simulink model "3DoFManipulatorWithBLDCM_SIMULATION"  (R2023b)
settings: Solver=VariableStepAuto  StartTime=0.0  StopTime=10  MaxStep=1e-4  RelTol=1e-3
undefined symbols (not defined in the file): X, Y, Z
libraries: spsMosfetLib x18, sm_lib x11, nesl_utility x7, eeGeneralControl x6, spsDCVoltageSourceLib x3, spsGroundLib x3, spsThreePhaseSeriesRLCBranchLib x3, spsThreePhaseVIMeasurementLib x3, slpidlib x3, sps_lib x1
(part 1 of 3)
settings Model: Creator=nicog  LastModifiedBy=nicog

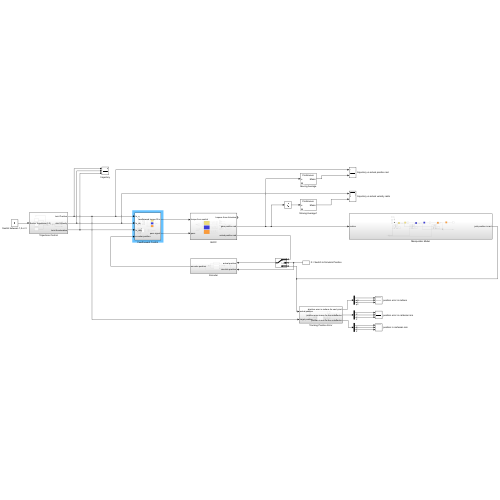
[thumbnail: Simulink's stored preview of the top-level diagram]
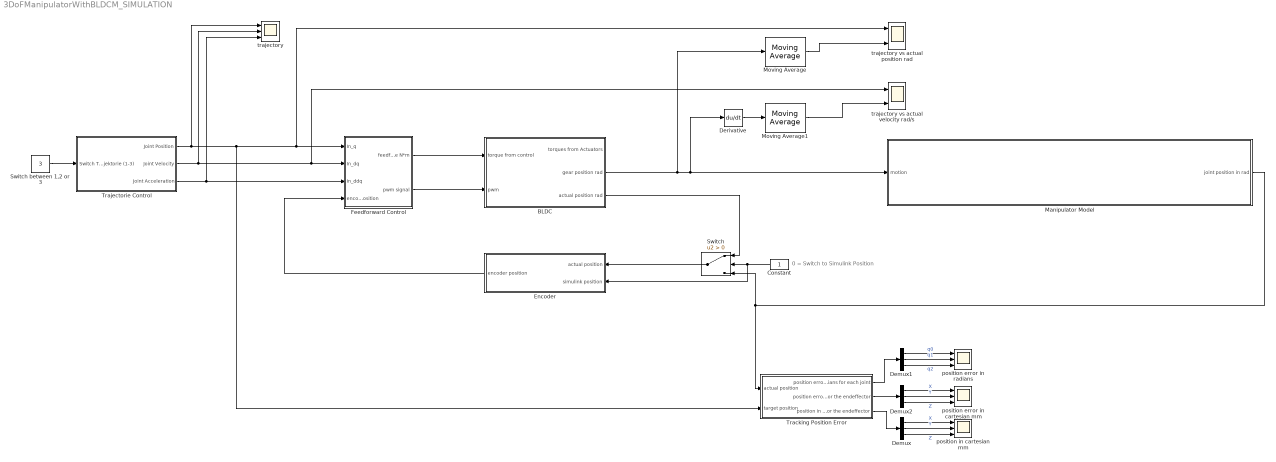
== system 3DoFManipulatorWithBLDCM_SIMULATION ==
  note: 0 = Switch to Simulink Position
  BLDC : Subsystem
  Constant : Constant
  Demux : Demux  Outputs=3
  Demux1 : Demux  Outputs=3
  Demux2 : Demux  Outputs=3
  Derivative : Derivative
  Encoder : Subsystem
  Feedforward Control : Subsystem
  Manipulator Model : Subsystem
  Moving Average : eeGeneralControl/Moving Average  VariantControl=Variant1  LabelModeActiveChoice=Continuous  f=60  x0=0  BufferSize=8192  Ts=0
      settings: LibrarySourceBlock=ee_sl_lib/General Control/Moving Average
  Moving Average1 : eeGeneralControl/Moving Average  VariantControl=Variant1  LabelModeActiveChoice=Continuous  f=60  x0=0  BufferSize=8192  Ts=0
      settings: LibrarySourceBlock=ee_sl_lib/General Control/Moving Average
  Switch : Switch  Criteria=u2 > Threshold  SaturateOnIntegerOverflow=off  InputSameDT=off
  Switch between 1,2 or 3 : Constant  Value=3
  Tracking Position Error : Subsystem
  Trajectorie Control : Subsystem
  position error in cartesian mm : Scope  NumInputPorts=3
  position error in radians : Scope  NumInputPorts=3
  position in cartesian mm : Scope  NumInputPorts=3
  trajectory : Scope  NumInputPorts=3
  trajectory vs actual position rad : Scope  NumInputPorts=2
  trajectory vs actual velocity rad/s : Scope  NumInputPorts=2
  wires:
  Trajectorie Control/2(Joint Velocity) -> trajectory/2, trajectory vs actual velocity rad/s/1, Feedforward Control/2(In_dq)
  Trajectorie Control/1(Joint Position) -> Tracking Position Error/2(target position), trajectory vs actual position rad/1, Feedforward Control/1(In_q), trajectory/1
  Trajectorie Control/3(Joint Acceleration) -> trajectory/3, Feedforward Control/3(In_ddq)
  Feedforward Control/1(feedforward torque N*m) -> BLDC/1(torque from control)
  Tracking Position Error/3(position in mm for the endeffector) -> Demux/1
  Switch between 1,2 or 3/1 -> Trajectorie Control/1(Switch Trajektorie (1-3))
  Demux/3 -> position in cartesian mm/3  "Z"
  Demux/2 -> position in cartesian mm/2  "Y"
  Demux/1 -> position in cartesian mm/1  "X"
  Tracking Position Error/1(position error in radians for each joint) -> Demux1/1
  Demux1/1 -> position error in radians/1  "q0"
  Demux1/2 -> position error in radians/2  "q1"
  Demux1/3 -> position error in radians/3  "q2"
  Demux2/1 -> position error in cartesian mm/1  "X"
  Demux2/2 -> position error in cartesian mm/2  "Y"
  Demux2/3 -> position error in cartesian mm/3  "Z"
  Tracking Position Error/2(position error in mm for the endeffector) -> Demux2/1
  BLDC/2(gear position rad) -> Moving Average/1, Derivative/1, Manipulator Model/1(motion)
  Switch/1 -> Encoder/1(actual position)
  Manipulator Model/1(joint position in rad) -> Tracking Position Error/1(actual position), Switch/3
  BLDC/3(actual position rad) -> Switch/1
  Constant/1 -> Encoder/2(simulink position), Switch/2
  Moving Average/1 -> trajectory vs actual position rad/2
  Moving Average1/1 -> trajectory vs actual velocity rad/s/2
  Derivative/1 -> Moving Average1/1
  Encoder/1(encoder position) -> Feedforward Control/4(encoder position)
  Feedforward Control/2(pwm signal) -> BLDC/2(pwm)

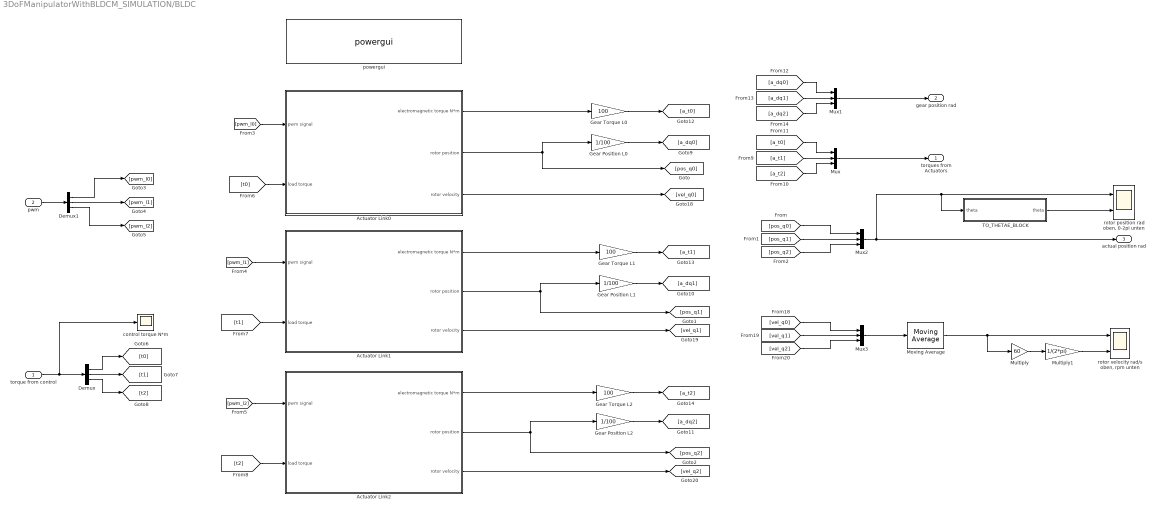
== system 3DoFManipulatorWithBLDCM_SIMULATION/BLDC ==
  torque from control : Inport
  pwm : Inport  Port=2
  Actuator Link0 : Subsystem
  Actuator Link1 : Subsystem
  Actuator Link2 : Subsystem
  Demux : Demux  Outputs=3
  Demux1 : Demux  Outputs=3
  Gear Position L0 : Gain  Gain=1/100
  Gear Position L1 : Gain  Gain=1/100
  Gear Position L2 : Gain  Gain=1/100
  Gear Torque L0 : Gain  Gain=100
  Gear Torque L1 : Gain  Gain=100
  Gear Torque L2 : Gain  Gain=100
  Moving Average : eeGeneralControl/Moving Average  VariantControl=Variant1  LabelModeActiveChoice=Continuous  f=30  x0=0  BufferSize=8192  Ts=0
      settings: LibrarySourceBlock=ee_sl_lib/General Control/Moving Average
  Multiply : Gain  Gain=60
  Multiply1 : Gain  Gain=1/(2*pi)
  Mux{,1..3} (4 alike) : Mux  Inputs=3
  TO_THETAE_BLOCK : MATLAB Function  TreatAsAtomicUnit=on
  control torque N*m : Scope
  powergui : sps_lib/powergui  Priority=1  SimulationMode=Discrete  SampleTime=1e-4  frequency=60  Iterations=50  frequencyindice=0  Pbase=100e6  ErrMax=1e-4  UnitsV=kV  UnitsW=MW  buscounter=0  FunctionMessages=off  echomessages=off  EnableUseOfTLC=off  CurrentSourceSwitches=off  DisableSnubberDevices=off  DisableRonSwitches=off  DisableVfSwitches=off  DisplayEquations=off  AutomaticDiscreteSolvers=off  SolverType=Tustin/Backward Euler (TBE)  Interpol=off  ExternalGateDelay=off  methode=off  Ts=100  x0status=blocks  SPID=on  SwTol=0  HookPort=off  NonlinearTolerance=1e-4  nMaxIteration=100  ContinueOnMaxIteration=off  RestoreLinks=warning  ResistiveCurrentMeasurement=off  Frange=[0:2:500]  Ylog=off  Xlog=on  ShowGrid=off  save=off  variable=ZData  structure=0  ZoomFFT=off  StartTime=0.0  cycles=1  DisplayStyle=1  fundamental=60  FreqAxis=off  MaxFrequency=1000  frequencyindicesteady=1  RmsSteady=1  display=off
  "rotor position rad oben, 0-2pi unten" : Scope  NumInputPorts=2
  "rotor velocity rad/s oben, rpm unten" : Scope  NumInputPorts=2
  torques from Actuators : Outport
  gear position rad : Outport  Port=2
  actual position rad : Outport  Port=3
  wires:
  torque from control/1 -> control torque N*m/1, Demux/1
  Actuator Link0/1(electromagnetic torque N*m) -> Gear Torque L0/1
  Actuator Link1/1(electromagnetic torque N*m) -> Gear Torque L1/1
  Actuator Link2/1(electromagnetic torque N*m) -> Gear Torque L2/1
  Mux1/1 -> gear position rad/1
  Mux2/1 -> TO_THETAE_BLOCK/1("theta "), "rotor position rad oben, 0-2pi unten"/1, actual position rad/1
  Mux/1 -> torques from Actuators/1
  Actuator Link0/2(rotor position) -> [pos_q0], Gear Position L0/1
  Actuator Link1/2(rotor position) -> [pos_q1], Gear Position L1/1
  Actuator Link2/2(rotor position) -> [pos_q2], Gear Position L2/1
  [pos_q0] -> Mux2/1
  [pos_q1] -> Mux2/2
  [pos_q2] -> Mux2/3
  Demux/1 -> [t0]
  Demux/2 -> [t1]
  Demux/3 -> [t2]
  [t0] -> Actuator Link0/2(load torque)
  Gear Position L0/1 -> [a_dq0]
  Gear Position L1/1 -> [a_dq1]
  Gear Position L2/1 -> [a_dq2]
  Gear Torque L0/1 -> [a_t0]
  Gear Torque L1/1 -> [a_t1]
  Gear Torque L2/1 -> [a_t2]
  [a_t0] -> Mux/1
  [a_t1] -> Mux/2
  [a_t2] -> Mux/3
  [a_dq0] -> Mux1/1
  [a_dq1] -> Mux1/2
  [a_dq2] -> Mux1/3
  [vel_q1] -> Mux3/2
  Mux3/1 -> Moving Average/1
  [vel_q2] -> Mux3/3
  [vel_q0] -> Mux3/1
  Multiply/1 -> Multiply1/1
  Moving Average/1 -> Multiply/1, "rotor velocity rad/s oben, rpm unten"/1
  Multiply1/1 -> "rotor velocity rad/s oben, rpm unten"/2
  TO_THETAE_BLOCK/1(theta) -> "rotor position rad oben, 0-2pi unten"/2
  Actuator Link0/3(rotor velocity) -> [vel_q0]
  Actuator Link1/3(rotor velocity) -> [vel_q1]
  Actuator Link2/3(rotor velocity) -> [vel_q2]
  [t1] -> Actuator Link1/2(load torque)
  pwm/1 -> Demux1/1
  Demux1/1 -> [pwm_l0]
  Demux1/2 -> [pwm_l1]
  Demux1/3 -> [pwm_l2]
  [pwm_l0] -> Actuator Link0/1(pwm signal)
  [pwm_l1] -> Actuator Link1/1(pwm signal)
  [pwm_l2] -> Actuator Link2/1(pwm signal)
  [t2] -> Actuator Link2/2(load torque)

== system 3DoFManipulatorWithBLDCM_SIMULATION/Encoder ==
  actual position : Inport
  simulink position : Inport  Port=2
  Demux : Demux  Outputs=3
  ENCODER_BLOCK_L0 : MATLAB Function  TreatAsAtomicUnit=on  SystemSampleTime=1e-4
  ENCODER_BLOCK_L1 : MATLAB Function  TreatAsAtomicUnit=on  SystemSampleTime=1e-4
  ENCODER_BLOCK_L2 : MATLAB Function  TreatAsAtomicUnit=on  SystemSampleTime=1e-4
  Mux : Mux  Inputs=3
  Switch : Switch  Criteria=u2 > Threshold  SaturateOnIntegerOverflow=off  InputSameDT=off
  encoder position : Outport
  wires:
  Demux/1 -> ENCODER_BLOCK_L0/1(actual_position)
  Demux/2 -> ENCODER_BLOCK_L1/1(actual_position)
  Demux/3 -> ENCODER_BLOCK_L2/1(actual_position)
  ENCODER_BLOCK_L1/1(encoder_output) -> Mux/2
  ENCODER_BLOCK_L2/1(encoder_output) -> Mux/3
  ENCODER_BLOCK_L0/1(encoder_output) -> Mux/1
  simulink position/1 -> Switch/2
  Mux/1 -> Switch/1
  actual position/1 -> Demux/1, Switch/3
  Switch/1 -> encoder position/1

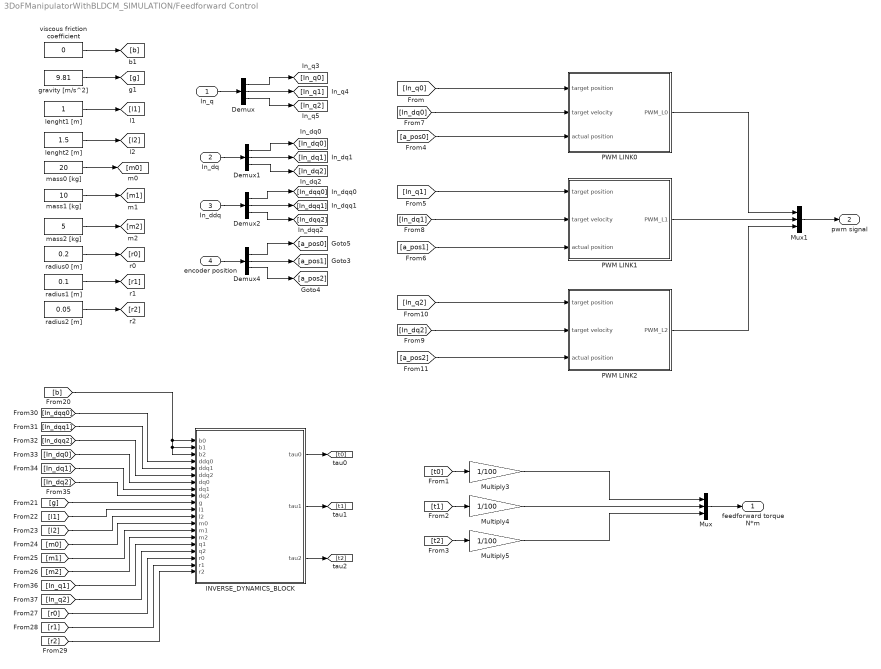
== system 3DoFManipulatorWithBLDCM_SIMULATION/Feedforward Control ==
  In_q : Inport
  In_dq : Inport  Port=2
  In_ddq : Inport  Port=3
  encoder position : Inport  Port=4
  Demux{,1..2,4} (4 alike) : Demux  Outputs=3
  INVERSE_DYNAMICS_BLOCK : MATLAB Function  TreatAsAtomicUnit=on
  Multiply3 : Gain  Gain=1/100
  Multiply4 : Gain  Gain=1/100
  Multiply5 : Gain  Gain=1/100
  Mux : Mux  Inputs=3
  Mux1 : Mux  Inputs=3
  PWM LINK0 : Subsystem
  PWM LINK1 : Subsystem
  PWM LINK2 : Subsystem
  "gravity [m/s^2] " : Constant  Value=9.81
  lenght1 [m] : Constant
  lenght2 [m] : Constant  Value=1.5
  mass0 [kg] : Constant  Value=20
  mass1 [kg] : Constant  Value=10
  mass2 [kg] : Constant  Value=5
  radius0 [m] : Constant  Value=0.2
  radius1 [m] : Constant  Value=0.1
  radius2 [m] : Constant  Value=0.05
  viscous friction coefficient : Constant  Value=0
  feedforward torque N*m : Outport
  pwm signal : Outport  Port=2
  wires:
  [r2] -> INVERSE_DYNAMICS_BLOCK/20(r2)
  [g] -> INVERSE_DYNAMICS_BLOCK/10(g)
  [r0] -> INVERSE_DYNAMICS_BLOCK/18(r0)
  [b] -> INVERSE_DYNAMICS_BLOCK/2(b1), INVERSE_DYNAMICS_BLOCK/3(b2), INVERSE_DYNAMICS_BLOCK/1(b0)
  [l1] -> INVERSE_DYNAMICS_BLOCK/11(l1)
  [m1] -> INVERSE_DYNAMICS_BLOCK/14(m1)
  [m2] -> INVERSE_DYNAMICS_BLOCK/15(m2)
  [m0] -> INVERSE_DYNAMICS_BLOCK/13(m0)
  [r1] -> INVERSE_DYNAMICS_BLOCK/19(r1)
  [l2] -> INVERSE_DYNAMICS_BLOCK/12(l2)
  In_q/1 -> Demux/1
  In_dq/1 -> Demux1/1
  In_ddq/1 -> Demux2/1
  Mux/1 -> feedforward torque N*m/1
  radius0 [m]/1 -> [r0]
  radius2 [m]/1 -> [r2]
  lenght2 [m]/1 -> [l2]
  viscous friction coefficient/1 -> [b]
  radius1 [m]/1 -> [r1]
  lenght1 [m]/1 -> [l1]
  mass0 [kg]/1 -> [m0]
  mass1 [kg]/1 -> [m1]
  mass2 [kg]/1 -> [m2]
  "gravity [m/s^2] "/1 -> [g]
  INVERSE_DYNAMICS_BLOCK/3(tau2) -> [t2]
  [t0] -> Multiply3/1
  [t1] -> Multiply4/1
  [t2] -> Multiply5/1
  Demux2/1 -> [In_dqq0]
  Demux2/2 -> [In_dqq1]
  Demux2/3 -> [In_dqq2]
  Demux1/2 -> [In_dq1]
  Demux1/1 -> [In_dq0]
  Demux1/3 -> [In_dq2]
  Demux/2 -> [In_q1]
  Demux/1 -> [In_q0]
  Demux/3 -> [In_q2]
  [In_dqq0] -> INVERSE_DYNAMICS_BLOCK/4(ddq0)
  [In_dqq1] -> INVERSE_DYNAMICS_BLOCK/5(ddq1)
  [In_dqq2] -> INVERSE_DYNAMICS_BLOCK/6(ddq2)
  [In_dq0] -> INVERSE_DYNAMICS_BLOCK/7(dq0)
  [In_dq1] -> INVERSE_DYNAMICS_BLOCK/8(dq1)
  [In_dq2] -> INVERSE_DYNAMICS_BLOCK/9(dq2)
  [In_q1] -> INVERSE_DYNAMICS_BLOCK/16(q1)
  [In_q2] -> INVERSE_DYNAMICS_BLOCK/17(q2)
  INVERSE_DYNAMICS_BLOCK/2(tau1) -> [t1]
  INVERSE_DYNAMICS_BLOCK/1(tau0) -> [t0]
  Multiply3/1 -> Mux/1
  Multiply4/1 -> Mux/2
  Multiply5/1 -> Mux/3
  PWM LINK0/1(PWM_L0) -> Mux1/1
  Mux1/1 -> pwm signal/1
  [In_q1] -> PWM LINK1/1(target position)
  PWM LINK1/1(PWM_L1) -> Mux1/2
  [a_pos1] -> PWM LINK1/3(actual position)
  [a_pos0] -> PWM LINK0/3(actual position)
  Demux4/2 -> [a_pos1]
  [In_q0] -> PWM LINK0/1(target position)
  Demux4/3 -> [a_pos2]
  [a_pos2] -> PWM LINK2/3(actual position)
  Demux4/1 -> [a_pos0]
  [In_q2] -> PWM LINK2/1(target position)
  encoder position/1 -> Demux4/1
  PWM LINK2/1(PWM_L2) -> Mux1/3
  [In_dq0] -> PWM LINK0/2(target velocity)
  [In_dq1] -> PWM LINK1/2(target velocity)
  [In_dq2] -> PWM LINK2/2(target velocity)

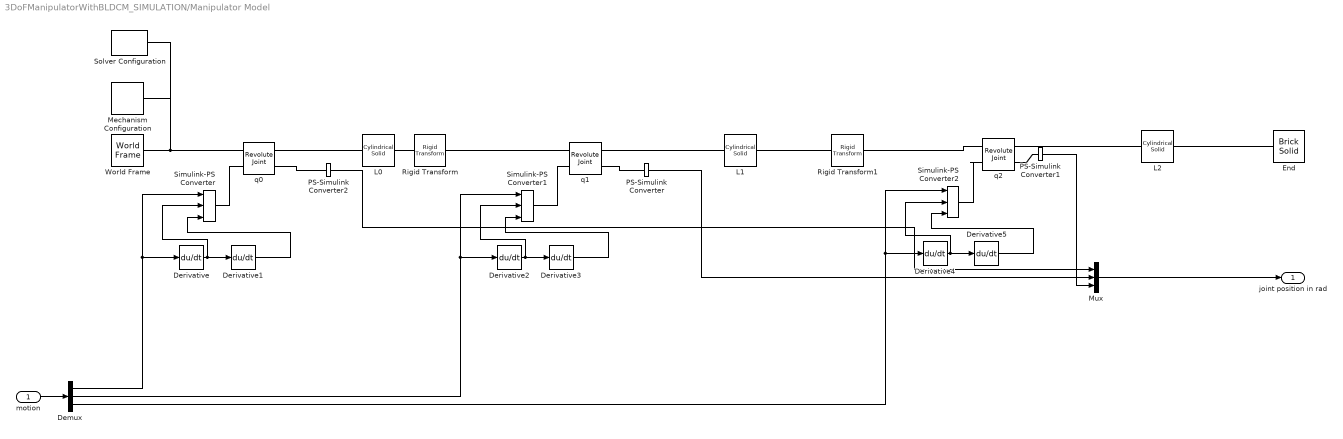
== system 3DoFManipulatorWithBLDCM_SIMULATION/Manipulator Model ==
  motion : Inport
  " L1" : sm_lib/Body Elements/Cylindrical Solid  GraphicAmbientColor=[0.15 0.15 0.15 1.0]  BasedOnType=Density  CenterOfMass=[0 0 0]  CenterOfMassUnits=m  GraphicDiffuseColor=[0.0 0.0 1.0]  CylinderLength=1  CylinderLengthUnits=m  CylinderRadius=0.1  CylinderRadiusUnits=m  Density=1000  DensityUnits=kg/m^3  DoExposeReferenceFrame=off  GraphicEmissiveColor=[0.0 0.0 0.0 1.0]  ExportEntireGeometry=off  SerializedFrames=<Frames><Frame><Id>Frame1</Id><Value><Name>F1</Name><Origin><Source>GeometricFeature</Source><FeatureName>bottom surface</FeatureName></Origin><PrimaryAxis><DefinedDirection>+X</DefinedDirection><Source>ReferenceFrame</Source><SourceDirection>+Z</SourceDirection><FeatureName></FeatureName></PrimaryAxis><SecondaryAxis><DefinedDirection>+Y</DefinedDirection><Source>ReferenceFrame</Source><SourceDirection>+X</SourceDirection><FeatureName></FeatureName></SecondaryAxis></Value></Frame><Frame><Id>Frame2</Id><Value><Name>F2</Name><Origin><Source>GeometricFeature</Source><FeatureName>top surface</FeatureName></Origin><PrimaryAxis><DefinedDirection>+X</DefinedDirection><Source>ReferenceFrame</Source><SourceDirection>+Z</SourceDirection><FeatureName></FeatureName></PrimaryAxis><SecondaryAxis><DefinedDirection>+Y</DefinedDirection><Source>ReferenceFrame</Source><SourceDirection>+X</SourceDirection><FeatureName></FeatureName></SecondaryAxis></Value></Frame></Frames>  MarkerShape=Sphere  MarkerSize=10  GraphicType=FromGeometry  InertiaType=PointMass  Mass=10  MassUnits=kg  MomentsOfInertia=[1 1 1]  MomentsOfInertiaUnits=kg*m^2  GraphicOpacity=1.0  ProductsOfInertia=[0 0 0]  ProductsOfInertiaUnits=kg*m^2  GraphicShininess=75  GraphicSpecularColor=[0.5 0.5 0.5 1.0]  GraphicVisPropType=SimpleVisualProperties
  Demux : Demux  Outputs=3
  Derivative{,1..5} (6 alike) : Derivative
  End : sm_lib/Body Elements/Brick Solid  GraphicAmbientColor=[0.15 0.15 0.15 1.0]  BasedOnType=Density  BrickDimensions=[1 1 1]  BrickDimensionsUnits=cm  CenterOfMass=[0 0 0]  CenterOfMassUnits=m  GraphicDiffuseColor=[1.0 0.0 0.4]  Density=1000  DensityUnits=kg/m^3  DoExposeReferenceFrame=on  GraphicEmissiveColor=[0.0 0.0 0.0 1.0]  ExportEntireGeometry=off  SerializedFrames=<Frames/>  MarkerShape=Sphere  MarkerSize=10  GraphicType=FromGeometry  InertiaType=PointMass  Mass=1  MassUnits=g  MomentsOfInertia=[1 1 1]  MomentsOfInertiaUnits=kg*m^2  GraphicOpacity=1.0  ProductsOfInertia=[0 0 0]  ProductsOfInertiaUnits=kg*m^2  GraphicShininess=75  GraphicSpecularColor=[0.5 0.5 0.5 1.0]  GraphicVisPropType=SimpleVisualProperties
  L0 : sm_lib/Body Elements/Cylindrical Solid  GraphicAmbientColor=[0.15 0.15 0.15 1.0]  BasedOnType=Density  CenterOfMass=[0 0 0]  CenterOfMassUnits=m  GraphicDiffuseColor=[1.0 1.0 0.0]  CylinderLength=0.5  CylinderLengthUnits=m  CylinderRadius=0.2  CylinderRadiusUnits=m  Density=1000  DensityUnits=kg/m^3  DoExposeReferenceFrame=off  GraphicEmissiveColor=[0.0 0.0 0.0 1.0]  ExportEntireGeometry=off  SerializedFrames=<Frames><Frame><Id>Frame1</Id><Value><Name>Bottom</Name><Origin><Source>GeometricFeature</Source><FeatureName>bottom surface</FeatureName></Origin><PrimaryAxis><DefinedDirection>+Z</DefinedDirection><Source>ReferenceFrame</Source><SourceDirection>+Z</SourceDirection><FeatureName></FeatureName></PrimaryAxis><SecondaryAxis><DefinedDirection>+X</DefinedDirection><Source>ReferenceFrame</Source><SourceDirection>+X</SourceDirection><FeatureName></FeatureName></SecondaryAxis></Value></Frame><Frame><Id>Frame2</Id><Value><Name>Top</Name><Origin><Source>GeometricFeature</Source><FeatureName>top surface</FeatureName></Origin><PrimaryAxis><DefinedDirection>+Z</DefinedDirection><Source>ReferenceFrame</Source><SourceDirection>+Z</SourceDirection><FeatureName></FeatureName></PrimaryAxis><SecondaryAxis><DefinedDirection>+X</DefinedDirection><Source>ReferenceFrame</Source><SourceDirection>+X</SourceDirection><FeatureName></FeatureName></SecondaryAxis></Value></Frame></Frames>  MarkerShape=Sphere  MarkerSize=10  GraphicType=FromGeometry  InertiaType=PointMass  Mass=20  MassUnits=kg  MomentsOfInertia=[1 1 1]  MomentsOfInertiaUnits=kg*m^2  GraphicOpacity=1.0  ProductsOfInertia=[0 0 0]  ProductsOfInertiaUnits=kg*m^2  GraphicShininess=75  GraphicSpecularColor=[0.5 0.5 0.5 1.0]  GraphicVisPropType=SimpleVisualProperties
  L2 : sm_lib/Body Elements/Cylindrical Solid  GraphicAmbientColor=[0.15 0.15 0.15 1.0]  BasedOnType=Density  CenterOfMass=[0 0 0]  CenterOfMassUnits=m  GraphicDiffuseColor=[1.0 0.6 0.0]  CylinderLength=1.5  CylinderLengthUnits=m  CylinderRadius=0.05  CylinderRadiusUnits=m  Density=1000  DensityUnits=kg/m^3  DoExposeReferenceFrame=off  GraphicEmissiveColor=[0.0 0.0 0.0 1.0]  ExportEntireGeometry=off  SerializedFrames=<Frames><Frame><Id>Frame1</Id><Value><Name>F1</Name><Origin><Source>GeometricFeature</Source><FeatureName>bottom surface</FeatureName></Origin><PrimaryAxis><DefinedDirection>+X</DefinedDirection><Source>ReferenceFrame</Source><SourceDirection>+Z</SourceDirection><FeatureName></FeatureName></PrimaryAxis><SecondaryAxis><DefinedDirection>+Y</DefinedDirection><Source>ReferenceFrame</Source><SourceDirection>+X</SourceDirection><FeatureName></FeatureName></SecondaryAxis></Value></Frame><Frame><Id>Frame2</Id><Value><Name>F2</Name><Origin><Source>GeometricFeature</Source><FeatureName>top surface</FeatureName></Origin><PrimaryAxis><DefinedDirection>+X</DefinedDirection><Source>ReferenceFrame</Source><SourceDirection>+Z</SourceDirection><FeatureName></FeatureName></PrimaryAxis><SecondaryAxis><DefinedDirection>+Y</DefinedDirection><Source>ReferenceFrame</Source><SourceDirection>+X</SourceDirection><FeatureName></FeatureName></SecondaryAxis></Value></Frame></Frames>  MarkerShape=Sphere  MarkerSize=10  GraphicType=FromGeometry  InertiaType=PointMass  Mass=5  MassUnits=kg  MomentsOfInertia=[1 1 1]  MomentsOfInertiaUnits=kg*m^2  GraphicOpacity=1.0  ProductsOfInertia=[0 0 0]  ProductsOfInertiaUnits=kg*m^2  GraphicShininess=75  GraphicSpecularColor=[0.5 0.5 0.5 1.0]  GraphicVisPropType=SimpleVisualProperties
  Mechanism Configuration : sm_lib/Utilities/Mechanism Configuration  UniformGravity=Constant  GravityVector=[0 0 -9.80665]  GravityVectorUnits=m/s^2  LinearizationDelta=0.001  JointModeTransitionNonlinearIterations=2
  Mux : Mux  Inputs=3
  PS-Simulink Converter : nesl_utility/PS-Simulink Converter  PhysicalDomain=network_engine_domain  SubClassName=ps_output  LeftPortType=input  RightPortType=output  PseudoPeriodic=off  Frequencies=[]  VectorFormat=inherit  Unit=inherit  AffineConversion=off
  PS-Simulink Converter1 : nesl_utility/PS-Simulink Converter  PhysicalDomain=network_engine_domain  SubClassName=ps_output  LeftPortType=input  RightPortType=output  PseudoPeriodic=off  Frequencies=[]  VectorFormat=inherit  Unit=inherit  AffineConversion=off
  PS-Simulink Converter2 : nesl_utility/PS-Simulink Converter  PhysicalDomain=network_engine_domain  SubClassName=ps_output  LeftPortType=input  RightPortType=output  PseudoPeriodic=off  Frequencies=[]  VectorFormat=inherit  Unit=inherit  AffineConversion=off
  Rigid Transform : sm_lib/Frames and Transforms/Rigid Transform  TranslationMethod=None  TranslationStandardOffset=0  TranslationStandardOffsetUnits=m  TranslationStandardAxis=+Z  TranslationCartesianOffset=[0 0 0]  TranslationCartesianOffsetUnits=m  TranslationROffset=0  TranslationROffsetUnits=m  TranslationZOffset=0  TranslationZOffsetUnits=m  TranslationThetaOffset=0  TranslationThetaOffsetUnits=deg  RotationMethod=RotationSequence  RotationAngleUnits=rad  RotationStandardAxis=+X  RotationAngle=pi/2  RotationArbitraryAxis=[0 0 1]  FollAlignAxisA=+X  BaseAlignAxisA=+Y  FollAlignAxisB=+Y  BaseAlignAxisB=+Z  RotationSequenceAxes=FollowerAxes  RotationSequence=XZX  RotationSequenceAngles=[90 140 0]  RotationSequenceAnglesUnits=deg  RotationMatrix=[1 0 0; 0 1 0; 0 0 1]  Quaternion=[1 0 0 0]
  Rigid Transform1 : sm_lib/Frames and Transforms/Rigid Transform  TranslationMethod=None  TranslationStandardOffset=0  TranslationStandardOffsetUnits=m  TranslationStandardAxis=+Z  TranslationCartesianOffset=[0 0 0]  TranslationCartesianOffsetUnits=m  TranslationROffset=0  TranslationROffsetUnits=m  TranslationZOffset=0  TranslationZOffsetUnits=m  TranslationThetaOffset=0  TranslationThetaOffsetUnits=deg  RotationMethod=RotationSequence  RotationAngleUnits=rad  RotationStandardAxis=+X  RotationAngle=pi/2  RotationArbitraryAxis=[0 0 1]  FollAlignAxisA=+X  BaseAlignAxisA=+Y  FollAlignAxisB=+Y  BaseAlignAxisB=+Z  RotationSequenceAxes=FollowerAxes  RotationSequence=ZXY  RotationSequenceAngles=[-140 0 0]  RotationSequenceAnglesUnits=deg  RotationMatrix=[1 0 0; 0 1 0; 0 0 1]  Quaternion=[1 0 0 0]
  Simulink-PS Converter : nesl_utility/Simulink-PS Converter  PhysicalDomain=network_engine_domain  SubClassName=ps_input  LeftPortType=input  RightPortType=output  PseudoPeriodic=off  Frequencies=[]  NoiseDistribution=none  NoiseParameters=[]  Unit=rad  AffineConversion=off  FilteringAndDerivatives=provide  SimscapeFilterOrder=2  InputFilterTimeConstant=0.001  UdotUserProvided=2
  Simulink-PS Converter1 : nesl_utility/Simulink-PS Converter  PhysicalDomain=network_engine_domain  SubClassName=ps_input  LeftPortType=input  RightPortType=output  PseudoPeriodic=off  Frequencies=[]  NoiseDistribution=none  NoiseParameters=[]  Unit=rad  AffineConversion=off  FilteringAndDerivatives=provide  SimscapeFilterOrder=2  InputFilterTimeConstant=0.001  UdotUserProvided=2
  Simulink-PS Converter2 : nesl_utility/Simulink-PS Converter  PhysicalDomain=network_engine_domain  SubClassName=ps_input  LeftPortType=input  RightPortType=output  PseudoPeriodic=off  Frequencies=[]  NoiseDistribution=none  NoiseParameters=[]  Unit=rad  AffineConversion=off  FilteringAndDerivatives=provide  SimscapeFilterOrder=2  InputFilterTimeConstant=0.001  UdotUserProvided=2
  Solver Configuration : nesl_utility/Solver Configuration  PhysicalDomain=network_engine_domain  SubClassName=solver  LeftPortType=input  RightPortType=generic  Tones=[]  Harmonics=[]  SimulateNoise=off  Profile=off  UseLocalSampling=off  EnableSwitchedLinearOptims=on  FrequencyDomain=off  UseCCode=off  RelTol=0.001  AbsTol=0.001  MinStep=1e-09  ToWorkspace=off  RevertToSquareIcSolve=off  NumHomotopyIterations=100  PhasorMode=off  PhasorModeNumHarmonics=1  ConsistencySolver=NEWTON_XTOL_AFTER_FTOL  IndexReductionMethod=DerivativeReplacement  DoDC=off  ResidualTolerance=1e-09  ConsistencyTolSource=GLOBAL  ConsistencyAbsTol=0.001  ConsistencyRelTol=0.001  ConsistencyTolFactor=0.001  UseLocalSolver=off  LocalSolverChoice=NE_BACKWARD_EULER_ADVANCER  ResolveIndetEquations=on  FunctionEvalNumThread=1  LocalSolverSampleTime=0.001  DoFixedCost=off  MaxNonlinIter=3  MaxModeIter=2  ComputeImpulses=off  ImpulseIterations=2  LinearAlgebra=auto  LinearAlgebraNumThread=0  EquationFormulation=NE_TIME_EF  DelaysMemoryBudget=1024  AutomaticFiltering=on  FilteringTimeConstant=0.001  PartitionStorageMethod=AS_NEEDED  PartitionMemoryBudget=1024  PartitionMethod=ROBUST  MultibodyUseLocalSolver=off  MultibodyLocalSolverChoice=ODE1  MultibodyLocalSolverSampleTime=0.001
  World Frame : sm_lib/Frames and Transforms/World Frame
  q0 : sm_lib/Joints/Revolute Joint  JointMode=Normal  SenseConstraintForce=off  SenseConstraintForceX=off  SenseConstraintForceY=off  SenseConstraintForceZ=off  SenseConstraintTorque=off  SenseConstraintTorqueX=off  SenseConstraintTorqueY=off  SenseConstraintTorqueZ=off  SenseTotalForce=off  SenseTotalForceX=off  SenseTotalForceY=off  SenseTotalForceZ=off  SenseTotalTorque=off  SenseTotalTorqueX=off  SenseTotalTorqueY=off  SenseTotalTorqueZ=off  CompositeWrenchDir=FollowerOnBase  CompositeWrenchFrame=BaseFrame  EquilibriumPosition=0  EquilibriumPositionUnits=deg  SpringStiffness=0  SpringStiffnessUnits=N*m/deg  DampingCoefficient=0  DampingCoefficientUnits=N*m/(deg/s)  TorqueActuationMode=ComputedTorque  MotionActuationMode=InputMotion  SensePosition=on  SenseVelocity=off  SenseAcceleration=off  SenseTorqueForce=off  SenseLowerLimitTorqueForce=off  SenseUpperLimitTorqueForce=off  LowerLimitSpecify=on  LowerLimitBound=-180  LowerLimitBoundUnits=deg  LowerLimitStiffness=1e4  LowerLimitStiffnessUnits=N*m/deg  LowerLimitDamping=10  LowerLimitDampingUnits=N*m/(deg/s)  LowerLimitTransitionRegionWidth=0.1  LowerLimitTransitionRegionWidthUnits=deg  UpperLimitSpecify=on  UpperLimitBound=180  UpperLimitBoundUnits=deg  UpperLimitStiffness=1e4  UpperLimitStiffnessUnits=N*m/deg  UpperLimitDamping=10  UpperLimitDampingUnits=N*m/(deg/s)  UpperLimitTransitionRegionWidth=0.1  UpperLimitTransitionRegionWidthUnits=deg  PositionTargetSpecify=off  PositionTargetPriority=High  PositionTargetValue=0  PositionTargetValueUnits=deg  VelocityTargetSpecify=off  VelocityTargetPriority=High  VelocityTargetValue=0  VelocityTargetValueUnits=deg/s
  q1 : sm_lib/Joints/Revolute Joint  JointMode=Normal  SenseConstraintForce=off  SenseConstraintForceX=off  SenseConstraintForceY=off  SenseConstraintForceZ=off  SenseConstraintTorque=off  SenseConstraintTorqueX=off  SenseConstraintTorqueY=off  SenseConstraintTorqueZ=off  SenseTotalForce=off  SenseTotalForceX=off  SenseTotalForceY=off  SenseTotalForceZ=off  SenseTotalTorque=off  SenseTotalTorqueX=off  SenseTotalTorqueY=off  SenseTotalTorqueZ=off  CompositeWrenchDir=FollowerOnBase  CompositeWrenchFrame=BaseFrame  EquilibriumPosition=0  EquilibriumPositionUnits=deg  SpringStiffness=0  SpringStiffnessUnits=N*m/deg  DampingCoefficient=0  DampingCoefficientUnits=N*m/(deg/s)  TorqueActuationMode=ComputedTorque  MotionActuationMode=InputMotion  SensePosition=on  SenseVelocity=off  SenseAcceleration=off  SenseTorqueForce=off  SenseLowerLimitTorqueForce=off  SenseUpperLimitTorqueForce=off  LowerLimitSpecify=on  LowerLimitBound=-120  LowerLimitBoundUnits=deg  LowerLimitStiffness=1e4  LowerLimitStiffnessUnits=N*m/deg  LowerLimitDamping=10  LowerLimitDampingUnits=N*m/(deg/s)  LowerLimitTransitionRegionWidth=0.1  LowerLimitTransitionRegionWidthUnits=deg  UpperLimitSpecify=on  UpperLimitBound=0  UpperLimitBoundUnits=deg  UpperLimitStiffness=1e4  UpperLimitStiffnessUnits=N*m/deg  UpperLimitDamping=10  UpperLimitDampingUnits=N*m/(deg/s)  UpperLimitTransitionRegionWidth=0.1  UpperLimitTransitionRegionWidthUnits=deg  PositionTargetSpecify=off  PositionTargetPriority=High  PositionTargetValue=0  PositionTargetValueUnits=deg  VelocityTargetSpecify=off  VelocityTargetPriority=High  VelocityTargetValue=0  VelocityTargetValueUnits=deg/s
  q2 : sm_lib/Joints/Revolute Joint  JointMode=Normal  SenseConstraintForce=off  SenseConstraintForceX=off  SenseConstraintForceY=off  SenseConstraintForceZ=off  SenseConstraintTorque=off  SenseConstraintTorqueX=off  SenseConstraintTorqueY=off  SenseConstraintTorqueZ=off  SenseTotalForce=off  SenseTotalForceX=off  SenseTotalForceY=off  SenseTotalForceZ=off  SenseTotalTorque=off  SenseTotalTorqueX=off  SenseTotalTorqueY=off  SenseTotalTorqueZ=off  CompositeWrenchDir=FollowerOnBase  CompositeWrenchFrame=BaseFrame  EquilibriumPosition=0  EquilibriumPositionUnits=deg  SpringStiffness=0  SpringStiffnessUnits=N*m/deg  DampingCoefficient=0  DampingCoefficientUnits=N*m/(deg/s)  TorqueActuationMode=ComputedTorque  MotionActuationMode=InputMotion  SensePosition=on  SenseVelocity=off  SenseAcceleration=off  SenseTorqueForce=off  SenseLowerLimitTorqueForce=off  SenseUpperLimitTorqueForce=off  LowerLimitSpecify=on  LowerLimitBound=0  LowerLimitBoundUnits=deg  LowerLimitStiffness=1e4  LowerLimitStiffnessUnits=N*m/deg  LowerLimitDamping=10  LowerLimitDampingUnits=N*m/(deg/s)  LowerLimitTransitionRegionWidth=0.1  LowerLimitTransitionRegionWidthUnits=deg  UpperLimitSpecify=on  UpperLimitBound=140  UpperLimitBoundUnits=deg  UpperLimitStiffness=1e4  UpperLimitStiffnessUnits=N*m/deg  UpperLimitDamping=10  UpperLimitDampingUnits=N*m/(deg/s)  UpperLimitTransitionRegionWidth=0.1  UpperLimitTransitionRegionWidthUnits=deg  PositionTargetSpecify=off  PositionTargetPriority=High  PositionTargetValue=0  PositionTargetValueUnits=deg  VelocityTargetSpecify=off  VelocityTargetPriority=High  VelocityTargetValue=0  VelocityTargetValueUnits=deg/s
  joint position in rad : Outport
  wires:
  PS-Simulink Converter/1 -> Mux/2
  PS-Simulink Converter2/1 -> Mux/1
  Mux/1 -> joint position in rad/1
  Demux/1 -> Derivative/1, Simulink-PS Converter/1
  motion/1 -> Demux/1
  PS-Simulink Converter1/1 -> Mux/3
  Derivative/1 -> Simulink-PS Converter/2, Derivative1/1
  Derivative1/1 -> Simulink-PS Converter/3
  Demux/2 -> Derivative2/1, Simulink-PS Converter1/1
  Derivative2/1 -> Simulink-PS Converter1/2, Derivative3/1
  Derivative3/1 -> Simulink-PS Converter1/3
  Demux/3 -> Derivative4/1, Simulink-PS Converter2/1
  Derivative4/1 -> Simulink-PS Converter2/2, Derivative5/1
  Derivative5/1 -> Simulink-PS Converter2/3
  connections:
  PS-Simulink Converter2/LConn1 -- q0/RConn2
  " L1"/RConn1 -- Rigid Transform1/LConn1
  q1/LConn1 -- Rigid Transform/RConn1
  q0/RConn1 -- L0/LConn1
  World Frame/RConn1 -- Solver Configuration/RConn1 -- Mechanism Configuration/RConn1 -- q0/LConn1
  q2/RConn1 -- L2/LConn1
  " L1"/LConn1 -- q1/RConn1
  L0/RConn1 -- Rigid Transform/LConn1
  PS-Simulink Converter/LConn1 -- q1/RConn2
  L2/RConn1 -- End/RConn1
  Simulink-PS Converter1/RConn1 -- q1/LConn2
  q2/RConn2 -- PS-Simulink Converter1/LConn1
  q2/LConn2 -- Simulink-PS Converter2/RConn1
  q0/LConn2 -- Simulink-PS Converter/RConn1
  Rigid Transform1/RConn1 -- q2/LConn1

== system 3DoFManipulatorWithBLDCM_SIMULATION/Tracking Position Error ==
  actual position : Inport
  target position : Inport  Port=2
  Demux : Demux  Outputs=3
  Demux1 : Demux  Outputs=3
  Scope : Scope
  To Workspace : ToWorkspace  VariableName=positionCartesian  SaveFormat=Timeseries  SampleTime=-1
  To Workspace1 : ToWorkspace  VariableName=positionErrorRadians  SaveFormat=Timeseries  SampleTime=-1
  To Workspace2 : ToWorkspace  VariableName=positionErrorCartesian  SaveFormat=Timeseries  SampleTime=-1
  forward Kinematic : MATLAB Function  TreatAsAtomicUnit=on
  position error mm : Sum  Inputs=|+-
  position error rad : Sum  Inputs=|+-
  position error in radians for each joint : Outport
  position error in mm for the endeffector : Outport  Port=2
  position in mm for the endeffector : Outport  Port=3
  wires:
  actual position/1 -> Scope/1, Demux/1, position error rad/1
  target position/1 -> position error rad/2, Demux1/1
  position error rad/1 -> To Workspace1/1, position error in radians for each joint/1
  forward Kinematic/1(actualCartesianPosition) -> position error mm/1, To Workspace/1, position in mm for the endeffector/1
  position error mm/1 -> To Workspace2/1, position error in mm for the endeffector/1
  Demux/2 -> forward Kinematic/2(q1a)
  Demux/1 -> forward Kinematic/1(q0a)
  Demux/3 -> forward Kinematic/3(q2a)
  Demux1/2 -> forward Kinematic/5(q1t)
  Demux1/1 -> forward Kinematic/4(q0t)
  Demux1/3 -> forward Kinematic/6(q2t)
  forward Kinematic/2(targetCartesianPosition) -> position error mm/2

== system 3DoFManipulatorWithBLDCM_SIMULATION/Trajectorie Control ==
  Switch Trajektorie (1-3) : Inport
  Demux : Demux  Outputs=3
  Multiport Switch : MultiPortSwitch  SaturateOnIntegerOverflow=off  InputSameDT=off
  Subsystem : Subsystem
  Subsystem1 : Subsystem
  Subsystem2 : Subsystem
  Joint Position : Outport
  Joint Velocity : Outport  Port=2
  Joint Acceleration : Outport  Port=3
  wires:
  Subsystem/1(Trajektorie 1) -> Multiport Switch/2
  Subsystem1/1(Trajektorie 2) -> Multiport Switch/3
  Subsystem2/1(Trajektorie 3) -> Multiport Switch/4
  Switch Trajektorie (1-3)/1 -> Multiport Switch/1
  Multiport Switch/1 -> Demux/1
  Demux/1 -> Joint Position/1
  Demux/2 -> Joint Velocity/1
  Demux/3 -> Joint Acceleration/1

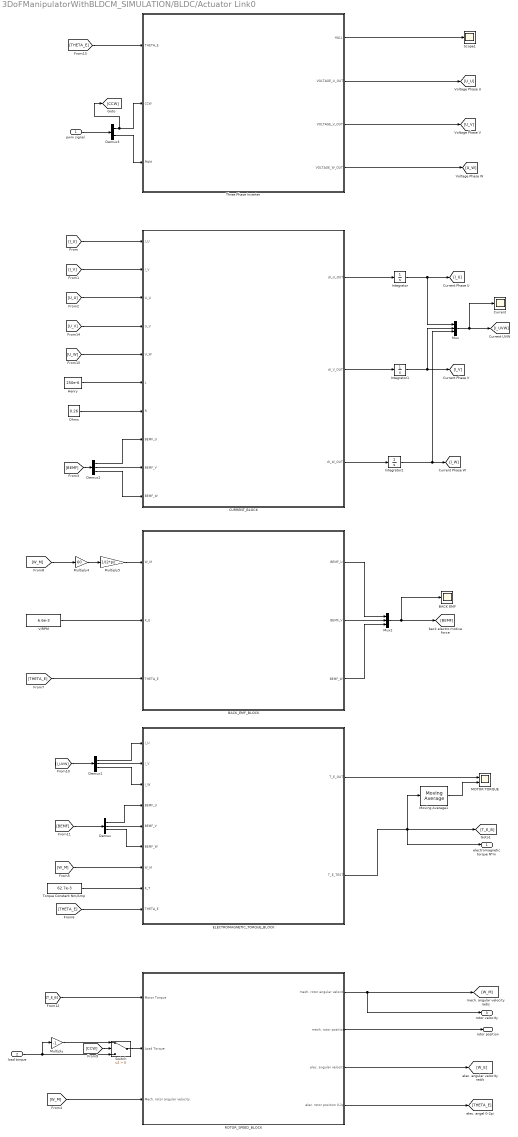
== system 3DoFManipulatorWithBLDCM_SIMULATION/BLDC/Actuator Link0 ==
  pwm signal : Inport
  load torque : Inport  Port=2
  BACK EMF : Scope
  BACK_EMF_BLOCK : MATLAB Function  TreatAsAtomicUnit=on
  CURRENT_BLOCK : MATLAB Function  TreatAsAtomicUnit=on
  Current : Scope
  Demux : Demux  Outputs=3
  Demux1 : Demux  Outputs=3
  Demux2 : Demux  Outputs=3
  Demux3 : Demux  Outputs=2
  ELECTROMAGNETIC_TORQUE_BLOCK : MATLAB Function  TreatAsAtomicUnit=on
  Henry : Constant  Value=250e-6
  Integrator : Integrator
  Integrator1 : Integrator
  Integrator2 : Integrator
  MOTOR TORQUE : Scope  NumInputPorts=2
  Moving Average1 : eeGeneralControl/Moving Average  VariantControl=Variant1  LabelModeActiveChoice=Continuous  f=30  x0=0  BufferSize=8192  Ts=0
      settings: LibrarySourceBlock=ee_sl_lib/General Control/Moving Average
  Multiply : Gain  Gain=-1
  Multiply4 : Gain  Gain=60
  Multiply5 : Gain  Gain=1/(2*pi)
  Mux : Mux  Inputs=3
  Mux2 : Mux  Inputs=3
  Ohms : Constant  Value=0.26
  ROTOR_SPEED_BLOCK : Subsystem
  Scope1 : Scope
  Switch : Switch  Criteria=u2 > Threshold  SaturateOnIntegerOverflow=off  InputSameDT=off
  Three Phase Inverter : Subsystem
  Torque Constant Nm/Amp : Constant  Value=62.7e-3
  V/RPM : Constant  Value=6.6e-3
  electromagnetic torque N*m : Outport
  rotor position : Outport  Port=2
  rotor velocity : Outport  Port=3
  wires:
  ELECTROMAGNETIC_TORQUE_BLOCK/2(T_E_TEST) -> Moving Average1/1, [T_E_B], electromagnetic torque N*m/1
  ELECTROMAGNETIC_TORQUE_BLOCK/1(T_E_OUT) -> MOTOR TORQUE/1
  Torque Constant Nm/Amp/1 -> ELECTROMAGNETIC_TORQUE_BLOCK/8(K_T)
  [I_V] -> CURRENT_BLOCK/2(I_V)
  [THETA_E] -> BACK_EMF_BLOCK/3(THETA_E)
  BACK_EMF_BLOCK/1(BEMF_U) -> Mux2/1
  Mux/1 -> Current/1, [I_UVW]
  Multiply5/1 -> BACK_EMF_BLOCK/1(W_M)
  Demux/3 -> ELECTROMAGNETIC_TORQUE_BLOCK/6(BEMF_W)
  Demux2/3 -> CURRENT_BLOCK/10(BEMF_W)
  V/RPM/1 -> BACK_EMF_BLOCK/2(K_E)
  Multiply4/1 -> Multiply5/1
  [BEMF] -> Demux2/1
  Demux2/1 -> CURRENT_BLOCK/8(BEMF_U)
  Demux2/2 -> CURRENT_BLOCK/9(BEMF_V)
  Integrator/1 -> [I_U], Mux/1
  [W_M] -> Multiply4/1
  [I_U] -> CURRENT_BLOCK/1(I_U)
  [THETA_E] -> ELECTROMAGNETIC_TORQUE_BLOCK/9(THETA_E)
  Mux2/1 -> BACK EMF/1, [BEMF]
  [U_W] -> CURRENT_BLOCK/5(U_W)
  [I_UVW] -> Demux1/1
  [U_U] -> CURRENT_BLOCK/3(U_U)
  Demux1/3 -> ELECTROMAGNETIC_TORQUE_BLOCK/3(I_W)
  BACK_EMF_BLOCK/2(BEMF_V) -> Mux2/2
  Demux1/2 -> ELECTROMAGNETIC_TORQUE_BLOCK/2(I_V)
  BACK_EMF_BLOCK/3(BEMF_W) -> Mux2/3
  Demux/2 -> ELECTROMAGNETIC_TORQUE_BLOCK/5(BEMF_V)
  Demux/1 -> ELECTROMAGNETIC_TORQUE_BLOCK/4(BEMF_U)
  [BEMF] -> Demux/1
  [U_V] -> CURRENT_BLOCK/4(U_V)
  CURRENT_BLOCK/1(dI_U_OUT) -> Integrator/1
  Integrator1/1 -> [I_V], Mux/2
  CURRENT_BLOCK/2(dI_V_OUT) -> Integrator1/1
  Integrator2/1 -> [I_W], Mux/3
  Ohms/1 -> CURRENT_BLOCK/7(R)
  [W_M] -> ELECTROMAGNETIC_TORQUE_BLOCK/7(W_M)
  CURRENT_BLOCK/3(dI_W_OUT) -> Integrator2/1
  Henry/1 -> CURRENT_BLOCK/6(L)
  Demux1/1 -> ELECTROMAGNETIC_TORQUE_BLOCK/1(I_U)
  Moving Average1/1 -> MOTOR TORQUE/2
  [THETA_E] -> Three Phase Inverter/1(THETA_E)
  Three Phase Inverter/1(HALL) -> Scope1/1
  Three Phase Inverter/3(VOLTAGE_V_OUT) -> [U_V]
  Three Phase Inverter/2(VOLTAGE_U_OUT) -> [U_U]
  Three Phase Inverter/4(VOLTAGE_W_OUT) -> [U_W]
  Demux3/1 -> [CCW], Three Phase Inverter/2(CCW)
  ROTOR_SPEED_BLOCK/1(mech. rotor angular velocity) -> [W_M], rotor velocity/1
  [T_E_B] -> ROTOR_SPEED_BLOCK/1(Motor Torque)
  [W_M] -> ROTOR_SPEED_BLOCK/3(Mech. rotor angular velocity)
  ROTOR_SPEED_BLOCK/2(mech. rotor position) -> rotor position/1
  ROTOR_SPEED_BLOCK/3(elec. angular velocity) -> [W_E]
  ROTOR_SPEED_BLOCK/4(elec. rotor position 0-2pi) -> [THETA_E]
  pwm signal/1 -> Demux3/1
  Demux3/2 -> Three Phase Inverter/3(PWM)
  [CCW] -> Switch/2
  Multiply/1 -> Switch/1
  load torque/1 -> Multiply/1, Switch/3
  Switch/1 -> ROTOR_SPEED_BLOCK/2(Load Torque)

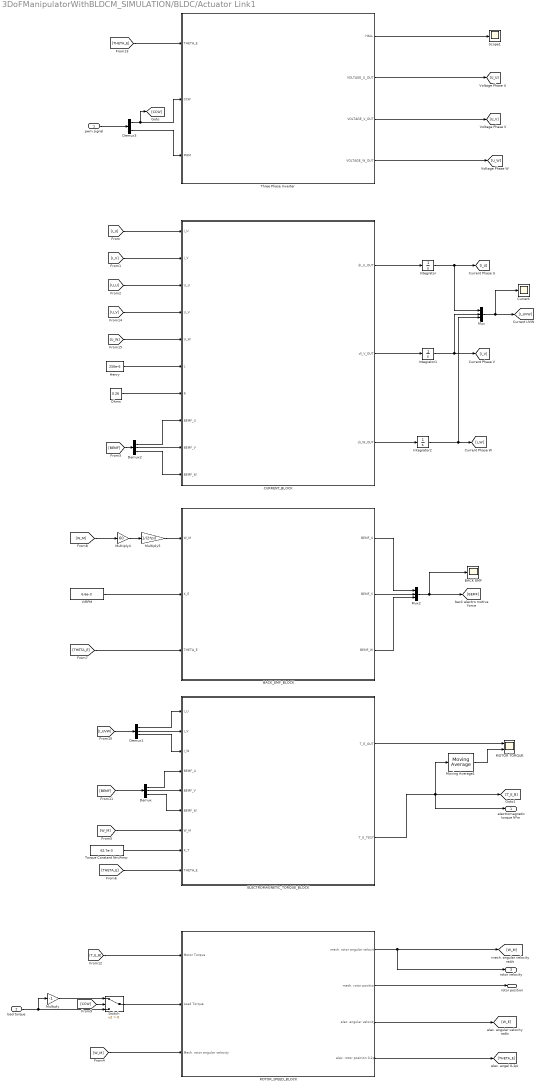
== system 3DoFManipulatorWithBLDCM_SIMULATION/BLDC/Actuator Link1 ==
  pwm signal : Inport
  load torque : Inport  Port=2
  BACK EMF : Scope
  BACK_EMF_BLOCK : MATLAB Function  TreatAsAtomicUnit=on
  CURRENT_BLOCK : MATLAB Function  TreatAsAtomicUnit=on
  Current : Scope
  Demux : Demux  Outputs=3
  Demux1 : Demux  Outputs=3
  Demux2 : Demux  Outputs=3
  Demux3 : Demux  Outputs=2
  ELECTROMAGNETIC_TORQUE_BLOCK : MATLAB Function  TreatAsAtomicUnit=on
  Henry : Constant  Value=250e-6
  Integrator : Integrator
  Integrator1 : Integrator
  Integrator2 : Integrator
  MOTOR TORQUE : Scope  NumInputPorts=2
  Moving Average1 : eeGeneralControl/Moving Average  VariantControl=Variant1  LabelModeActiveChoice=Continuous  f=30  x0=0  BufferSize=8192  Ts=0
      settings: LibrarySourceBlock=ee_sl_lib/General Control/Moving Average
  Multiply : Gain  Gain=-1
  Multiply4 : Gain  Gain=60
  Multiply5 : Gain  Gain=1/(2*pi)
  Mux : Mux  Inputs=3
  Mux2 : Mux  Inputs=3
  Ohms : Constant  Value=0.26
  ROTOR_SPEED_BLOCK : Subsystem
  Scope1 : Scope
  Switch : Switch  Criteria=u2 > Threshold  SaturateOnIntegerOverflow=off  InputSameDT=off
  Three Phase Inverter : Subsystem
  Torque Constant Nm/Amp : Constant  Value=62.7e-3
  V/RPM : Constant  Value=6.6e-3
  electromagnetic torque N*m : Outport
  rotor position : Outport  Port=2
  rotor velocity : Outport  Port=3
  wires:
  ELECTROMAGNETIC_TORQUE_BLOCK/2(T_E_TEST) -> Moving Average1/1, [T_E_B], electromagnetic torque N*m/1
  ELECTROMAGNETIC_TORQUE_BLOCK/1(T_E_OUT) -> MOTOR TORQUE/1
  Torque Constant Nm/Amp/1 -> ELECTROMAGNETIC_TORQUE_BLOCK/8(K_T)
  [I_V] -> CURRENT_BLOCK/2(I_V)
  [THETA_E] -> BACK_EMF_BLOCK/3(THETA_E)
  BACK_EMF_BLOCK/1(BEMF_U) -> Mux2/1
  Mux/1 -> Current/1, [I_UVW]
  Multiply5/1 -> BACK_EMF_BLOCK/1(W_M)
  Demux/3 -> ELECTROMAGNETIC_TORQUE_BLOCK/6(BEMF_W)
  Demux2/3 -> CURRENT_BLOCK/10(BEMF_W)
  V/RPM/1 -> BACK_EMF_BLOCK/2(K_E)
  Multiply4/1 -> Multiply5/1
  [BEMF] -> Demux2/1
  Demux2/1 -> CURRENT_BLOCK/8(BEMF_U)
  Demux2/2 -> CURRENT_BLOCK/9(BEMF_V)
  Integrator/1 -> [I_U], Mux/1
  [W_M] -> Multiply4/1
  [I_U] -> CURRENT_BLOCK/1(I_U)
  [THETA_E] -> ELECTROMAGNETIC_TORQUE_BLOCK/9(THETA_E)
  Mux2/1 -> BACK EMF/1, [BEMF]
  [U_W] -> CURRENT_BLOCK/5(U_W)
  [I_UVW] -> Demux1/1
  [U_U] -> CURRENT_BLOCK/3(U_U)
  Demux1/3 -> ELECTROMAGNETIC_TORQUE_BLOCK/3(I_W)
  BACK_EMF_BLOCK/2(BEMF_V) -> Mux2/2
  Demux1/2 -> ELECTROMAGNETIC_TORQUE_BLOCK/2(I_V)
  BACK_EMF_BLOCK/3(BEMF_W) -> Mux2/3
  Demux/2 -> ELECTROMAGNETIC_TORQUE_BLOCK/5(BEMF_V)
  Demux/1 -> ELECTROMAGNETIC_TORQUE_BLOCK/4(BEMF_U)
  [BEMF] -> Demux/1
  [U_V] -> CURRENT_BLOCK/4(U_V)
  CURRENT_BLOCK/1(dI_U_OUT) -> Integrator/1
  Integrator1/1 -> [I_V], Mux/2
  CURRENT_BLOCK/2(dI_V_OUT) -> Integrator1/1
  Integrator2/1 -> [I_W], Mux/3
  Ohms/1 -> CURRENT_BLOCK/7(R)
  [W_M] -> ELECTROMAGNETIC_TORQUE_BLOCK/7(W_M)
  CURRENT_BLOCK/3(dI_W_OUT) -> Integrator2/1
  Henry/1 -> CURRENT_BLOCK/6(L)
  Demux1/1 -> ELECTROMAGNETIC_TORQUE_BLOCK/1(I_U)
  Moving Average1/1 -> MOTOR TORQUE/2
  [THETA_E] -> Three Phase Inverter/1(THETA_E)
  Three Phase Inverter/1(HALL) -> Scope1/1
  Three Phase Inverter/3(VOLTAGE_V_OUT) -> [U_V]
  Three Phase Inverter/2(VOLTAGE_U_OUT) -> [U_U]
  Three Phase Inverter/4(VOLTAGE_W_OUT) -> [U_W]
  Demux3/1 -> Three Phase Inverter/2(CCW), [CCW]
  ROTOR_SPEED_BLOCK/1(mech. rotor angular velocity) -> [W_M], rotor velocity/1
  [T_E_B] -> ROTOR_SPEED_BLOCK/1(Motor Torque)
  [W_M] -> ROTOR_SPEED_BLOCK/3(Mech. rotor angular velocity)
  ROTOR_SPEED_BLOCK/2(mech. rotor position) -> rotor position/1
  ROTOR_SPEED_BLOCK/3(elec. angular velocity) -> [W_E]
  ROTOR_SPEED_BLOCK/4(elec. rotor position 0-2pi) -> [THETA_E]
  pwm signal/1 -> Demux3/1
  Demux3/2 -> Three Phase Inverter/3(PWM)
  Switch/1 -> ROTOR_SPEED_BLOCK/2(Load Torque)
  load torque/1 -> Multiply/1, Switch/3
  Multiply/1 -> Switch/1
  [CCW] -> Switch/2

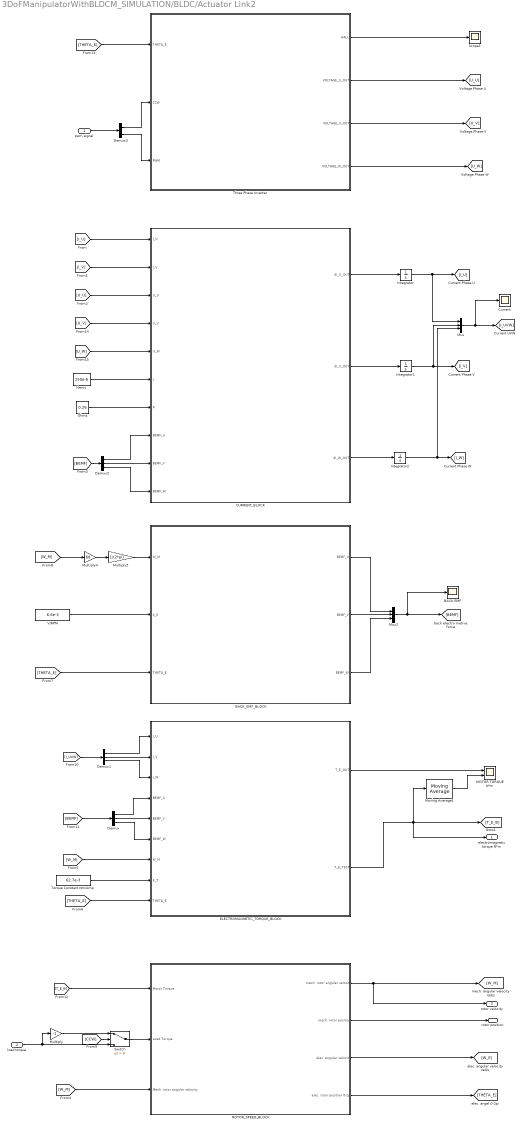
== system 3DoFManipulatorWithBLDCM_SIMULATION/BLDC/Actuator Link2 ==
  pwm signal : Inport
  load torque : Inport  Port=2
  BACK EMF : Scope
  BACK_EMF_BLOCK : MATLAB Function  TreatAsAtomicUnit=on
  CURRENT_BLOCK : MATLAB Function  TreatAsAtomicUnit=on
  Current : Scope
  Demux : Demux  Outputs=3
  Demux1 : Demux  Outputs=3
  Demux2 : Demux  Outputs=3
  Demux3 : Demux  Outputs=2
  ELECTROMAGNETIC_TORQUE_BLOCK : MATLAB Function  TreatAsAtomicUnit=on
  Henry : Constant  Value=250e-6
  Integrator : Integrator
  Integrator1 : Integrator
  Integrator2 : Integrator
  MOTOR TORQUE N*m : Scope  NumInputPorts=2
  Moving Average1 : eeGeneralControl/Moving Average  VariantControl=Variant1  LabelModeActiveChoice=Continuous  f=30  x0=0  BufferSize=8192  Ts=0
      settings: LibrarySourceBlock=ee_sl_lib/General Control/Moving Average
  Multiply : Gain  Gain=-1
  Multiply4 : Gain  Gain=60
  Multiply5 : Gain  Gain=1/(2*pi)
  Mux : Mux  Inputs=3
  Mux2 : Mux  Inputs=3
  Ohms : Constant  Value=0.26
  ROTOR_SPEED_BLOCK : Subsystem
  Scope1 : Scope
  Switch : Switch  Criteria=u2 > Threshold  SaturateOnIntegerOverflow=off  InputSameDT=off
  Three Phase Inverter : Subsystem
  Torque Constant Nm/Amp : Constant  Value=62.7e-3
  V/RPM : Constant  Value=6.6e-3
  electromagnetic torque N*m : Outport
  rotor position : Outport  Port=2
  rotor velocity : Outport  Port=3
  wires:
  ELECTROMAGNETIC_TORQUE_BLOCK/2(T_E_TEST) -> Moving Average1/1, [T_E_B], electromagnetic torque N*m/1
  ELECTROMAGNETIC_TORQUE_BLOCK/1(T_E_OUT) -> MOTOR TORQUE N*m/1
  Torque Constant Nm/Amp/1 -> ELECTROMAGNETIC_TORQUE_BLOCK/8(K_T)
  [I_V] -> CURRENT_BLOCK/2(I_V)
  [THETA_E] -> BACK_EMF_BLOCK/3(THETA_E)
  BACK_EMF_BLOCK/1(BEMF_U) -> Mux2/1
  Mux/1 -> Current/1, [I_UVW]
  Multiply5/1 -> BACK_EMF_BLOCK/1(W_M)
  Demux/3 -> ELECTROMAGNETIC_TORQUE_BLOCK/6(BEMF_W)
  Demux2/3 -> CURRENT_BLOCK/10(BEMF_W)
  V/RPM/1 -> BACK_EMF_BLOCK/2(K_E)
  Multiply4/1 -> Multiply5/1
  [BEMF] -> Demux2/1
  Demux2/1 -> CURRENT_BLOCK/8(BEMF_U)
  Demux2/2 -> CURRENT_BLOCK/9(BEMF_V)
  Integrator/1 -> [I_U], Mux/1
  [W_M] -> Multiply4/1
  [I_U] -> CURRENT_BLOCK/1(I_U)
  [THETA_E] -> ELECTROMAGNETIC_TORQUE_BLOCK/9(THETA_E)
  Mux2/1 -> BACK EMF/1, [BEMF]
  [U_W] -> CURRENT_BLOCK/5(U_W)
  [I_UVW] -> Demux1/1
  [U_U] -> CURRENT_BLOCK/3(U_U)
  Demux1/3 -> ELECTROMAGNETIC_TORQUE_BLOCK/3(I_W)
  BACK_EMF_BLOCK/2(BEMF_V) -> Mux2/2
  Demux1/2 -> ELECTROMAGNETIC_TORQUE_BLOCK/2(I_V)
  BACK_EMF_BLOCK/3(BEMF_W) -> Mux2/3
  Demux/2 -> ELECTROMAGNETIC_TORQUE_BLOCK/5(BEMF_V)
  Demux/1 -> ELECTROMAGNETIC_TORQUE_BLOCK/4(BEMF_U)
  [BEMF] -> Demux/1
  [U_V] -> CURRENT_BLOCK/4(U_V)
  CURRENT_BLOCK/1(dI_U_OUT) -> Integrator/1
  Integrator1/1 -> [I_V], Mux/2
  CURRENT_BLOCK/2(dI_V_OUT) -> Integrator1/1
  Integrator2/1 -> [I_W], Mux/3
  Ohms/1 -> CURRENT_BLOCK/7(R)
  [W_M] -> ELECTROMAGNETIC_TORQUE_BLOCK/7(W_M)
  CURRENT_BLOCK/3(dI_W_OUT) -> Integrator2/1
  Henry/1 -> CURRENT_BLOCK/6(L)
  Demux1/1 -> ELECTROMAGNETIC_TORQUE_BLOCK/1(I_U)
  Moving Average1/1 -> MOTOR TORQUE N*m/2
  [THETA_E] -> Three Phase Inverter/1(THETA_E)
  Three Phase Inverter/1(HALL) -> Scope1/1
  Three Phase Inverter/3(VOLTAGE_V_OUT) -> [U_V]
  Three Phase Inverter/2(VOLTAGE_U_OUT) -> [U_U]
  Three Phase Inverter/4(VOLTAGE_W_OUT) -> [U_W]
  Demux3/1 -> Three Phase Inverter/2(CCW)
  ROTOR_SPEED_BLOCK/1(mech. rotor angular velocity) -> [W_M], rotor velocity/1
  [T_E_B] -> ROTOR_SPEED_BLOCK/1(Motor Torque)
  [W_M] -> ROTOR_SPEED_BLOCK/3(Mech. rotor angular velocity)
  ROTOR_SPEED_BLOCK/2(mech. rotor position) -> rotor position/1
  ROTOR_SPEED_BLOCK/3(elec. angular velocity) -> [W_E]
  ROTOR_SPEED_BLOCK/4(elec. rotor position 0-2pi) -> [THETA_E]
  pwm signal/1 -> Demux3/1
  Demux3/2 -> Three Phase Inverter/3(PWM)
  [CCW] -> Switch/2
  Multiply/1 -> Switch/1
  load torque/1 -> Multiply/1, Switch/3
  Switch/1 -> ROTOR_SPEED_BLOCK/2(Load Torque)

== system 3DoFManipulatorWithBLDCM_SIMULATION/Feedforward Control/PWM LINK0 ==
  target position : Inport
  target velocity : Inport  Port=2
  actual position : Inport  Port=3
  CCW : Scope
  Duty Cycle : Scope
  Mux : Mux  Inputs=2
  PID Controller Position : slpidlib/PID Controller  Controller=PID  Form=Parallel  TimeDomain=Continuous-time  UseExternalTs=off  SampleTime=-1  IntegratorMethod=Forward Euler  FilterMethod=Forward Euler  ControllerParametersSource=internal  P=2000  I=15000  UseKiTs=off  D=0  N=100  UseFilter=on  TunerSelectOption=Transfer Function Based (PID Tuner App)  InitialConditionSource=internal  InitialConditionForIntegrator=0  InitialConditionForFilter=0  DifferentiatorICPrevScaledInput=0  ExternalReset=none  TrackingMode=off  Kt=1  LimitOutput=off  SatLimitsSource=internal  UpperSaturationLimit=inf  LowerSaturationLimit=-inf  LinearizeAsGain=on  AntiWindupMode=none  Kb=1  LimitIntegrator=off  UpperIntegratorSaturationLimit=inf  LowerIntegratorSaturationLimit=-inf  POutMin=[]  POutMax=[]  IOutMin=[]  IOutMax=[]  DOutMin=[]  DOutMax=[]  NOutMin=[]  NOutMax=[]  SumOutMin=[]  SumOutMax=[]  SaturationOutMin=[]  SaturationOutMax=[]  PParamMin=[]  PParamMax=[]  IParamMin=[]  IParamMax=[]  DParamMin=[]  DParamMax=[]  NParamMin=[]  NParamMax=[]  KbParamMin=[]  KbParamMax=[]  KtParamMin=[]  KtParamMax=[]  KbOutMin=[]  KbOutMax=[]  KtOutMin=[]  KtOutMax=[]  IntegratorOutMin=[]  IntegratorOutMax=[]  FilterOutMin=[]  FilterOutMax=[]  SumI1OutMin=[]  SumI1OutMax=[]  SumI2OutMin=[]  SumI2OutMax=[]  SumI3OutMin=[]  SumI3OutMax=[]  SumI4OutMin=[]  SumI4OutMax=[]  SumDOutMin=[]  SumDOutMax=[]  DifferentiatorOutMin=[]  DifferentiatorOutMax=[]  FilterDiffOutCoefMin=[]  FilterDiffOutCoefMax=[]  ReciprocalOutMin=[]  ReciprocalOutMax=[]  SumDenOutMin=[]  SumDenOutMax=[]  SumNumOutMin=[]  SumNumOutMax=[]  DivideOutMin=[]  DivideOutMax=[]  UdiffTsProdOutMin=[]  UdiffTsProdOutMax=[]  NTsProdOutMin=[]  NTsProdOutMax=[]  UintegralTsProdOutMin=[]  UintegralTsProdOutMax=[]  UngainTsProdOutMin=[]  UngainTsProdOutMax=[]  ClampingZeroOutDataTypeStr=Inherit: Inherit via back propagation  ClampingZeroOutMin=[]  ClampingZeroOutMax=[]  FilterDenConstantOutDataTypeStr=Inherit: Inherit via back propagation  FilterDenConstantOutMin=[]  FilterDenConstantOutMax=[]  PCopyOutDataTypeStr=Inherit: Inherit via back propagation  PCopyOutMin=[]  PCopyOutMax=[]  NCopyOutDataTypeStr=Inherit: Inherit via back propagation  NCopyOutMin=[]  NCopyOutMax=[]  IntegratorContinuousStateAttributes=''  IntegratorStateMustResolveToSignalObject=off  IntegratorRTWStateStorageClass=Auto  FilterContinuousStateAttributes=''  FilterStateMustResolveToSignalObject=off  FilterRTWStateStorageClass=Auto  ParallelPVariant=InternalParameters  IdealPVariant=Disabled  IVariant=InternalParameters  DVariant=InternalParameters  IntegratorVariant=Continuous  SatVariant=Disabled  AWVariant=Passthrough  PCopyVariant=Disabled  TRVariant=Disabled  FdbkBlocksVariant=Forward  IdealPFdbkVariant=Disabled  SatFdbkVariant=Disabled  DerivativeFilterVariant=ContFilter  NVariant=InternalParameters  NCopyVariant=Disabled  FilterICVariant=InternalICsFilter  IntegratorICVariant=InternalICs  ExternalResetVariant=Disabled  TRSumVariant=Passthrough  SumFdbkVariant=Disabled  SumVariant=Sum_PID  TsampFilterVariant=InternalTs  TsampNgainVariant=Passthrough  TsampIntegralVariant=Disabled_SignalSpec  ExternalSaturationOutDataTypeStr=Inherit: Same as second input
  PWM-Signal : Scope
  Variable Pulse Generator : VariablePulseGenerator  AllowZeroPulseWidth=on  SampleTime=0.1
  calculate duty cycle : MATLAB Function  TreatAsAtomicUnit=on
  diff_pos : MATLAB Function  TreatAsAtomicUnit=on  SystemSampleTime=1e-4
  PWM_L0 : Outport
  wires:
  Variable Pulse Generator/1 -> Mux/2, PWM-Signal/1
  [CCW] -> Mux/1
  target position/1 -> diff_pos/1(t_pos)
  calculate duty cycle/2(p) -> Variable Pulse Generator/2
  calculate duty cycle/1(dC) -> Duty Cycle/1, Variable Pulse Generator/1
  diff_pos/2(CCW) -> CCW/1, [CCW]
  Mux/1 -> PWM_L0/1
  diff_pos/1(diff_pos) -> PID Controller Position/1
  actual position/1 -> diff_pos/3(a_pos)
  PID Controller Position/1 -> calculate duty cycle/1(e_diff)
  target velocity/1 -> diff_pos/2(t_vel)
